simulink model "tut3"  (R2012b)
settings: Solver=ode45  StartTime=0.0  StopTime=8192  RelTol=1e-3
undefined symbols (not defined in the file): gcbh, pfb_coeff_gen_calc, xlBlockLoadCallback
libraries: xbsIndex_r4 x2165, casper_library_misc x93, casper_library_delays x38, xps_library x10, xbsReplacements_r4 x2, casper_library_pfbs x2, simulink x1, casper_library_ffts_twiddle x1, casper_library_reorder x1
(part 17 of 31)

== system tut3/fft_wideband_real/fft_direct/butterfly1_1/twiddle_general_4mult/coeff_gen ==
  rst : Inport
  Counter : xbsIndex_r4/Counter  cnt_type=Free Running  cnt_to=Inf  operation=Up  start_count=0  cnt_by_val=1  arith_type=Unsigned  n_bits=10  bin_pt=0  load_pin=off  rst=on  en=off  explicit_period=on  period=1  dbl_ovrd=off  use_behavioral_HDL=off  implementation=Fabric  block_type=counter
  ROM : xbsIndex_r4/ROM  depth=1024  initVector="[1                                      1                     0.9999847412109375                     0.9999542236328125                     0.9999237060546875                        0.9998779296875                     0.9998321533203125                     0.9997711181640625                       0.99969482421875                     0.9996185302734375                     0.9995269775390625                     0.9994354248046875                       0.99932861328125                       0.99920654296875                       0.99908447265625                     0.9989471435546875                     0.9987945556640625                     0.9986419677734375                       0.99847412109375                     0.9983062744140625                     0.9981231689453125                        0.9979248046875                     0.9977264404296875                     0.9975128173828125                      0.997283935546875                     0.9970550537109375                         0.996826171875                     0.9965667724609375                      0.996307373046875                     0.9960479736328125                     0.9957733154296875                        0.9954833984375                       0.99517822265625                         0.994873046875                       0.99456787109375                     0.9942474365234375                     0.9939117431640625                      0.993560791015625                     0.9932098388671875                     0.9928436279296875                     0.9924774169921875                      0.992095947265625                     0.9917144775390625                     0.9913177490234375                       0.99090576171875                         0.990478515625                       0.99005126953125                        0.9896240234375                     0.9891815185546875                     0.9887237548828125                      0.988250732421875                     0.9877777099609375                           0.9873046875                          0.98681640625                     0.9863128662109375                     0.9857940673828125                     0.9852752685546875                        0.9847412109375                     0.9842071533203125                     0.9836578369140625                     0.9831085205078125                        0.9825439453125                      0.981964111328125                       0.98138427734375                     0.9807891845703125                     0.9801788330078125                     0.9795684814453125                       0.97894287109375                     0.9783172607421875                     0.9776763916015625                     0.9770355224609375                     0.9763641357421875                        0.9757080078125                     0.9750213623046875                      0.974334716796875                     0.9736480712890625                     0.9729461669921875                       0.97222900390625                       0.97149658203125                     0.9707794189453125                       0.97003173828125                     0.9692840576171875                     0.9685211181640625                     0.9677581787109375                       0.96697998046875                        0.9661865234375                       0.96539306640625                     0.9645843505859375                      0.963775634765625                       0.96295166015625                      0.962127685546875                      0.961273193359375                     0.9604339599609375                      0.959564208984375                      0.958709716796875                       0.95782470703125                      0.956939697265625                     0.9560394287109375                       0.95513916015625                        0.9542236328125                       0.95330810546875                     0.9523773193359375                     0.9514312744140625 ...(+35900 chars)]"  distributed_mem=Block RAM  rst=off  init_reg=0  en=off  latency=2  gui_display_data_type=Fixed-point  arith_type="Signed  (2's comp)"  n_bits=18  bin_pt=16  preci_type=Single  exp_width=8  frac_width=24  dbl_ovrd=off  optimize=Area  use_rpm=on  block_type=sprom
  ROM1 : xbsIndex_r4/ROM  depth=1024  initVector="[0                    -0.0030670166015625                     -0.006134033203125                    -0.0092010498046875                      -0.01226806640625                    -0.0153350830078125                     -0.018402099609375                    -0.0214691162109375                       -0.0245361328125                    -0.0276031494140625                     -0.030670166015625                    -0.0337371826171875                      -0.03680419921875                    -0.0398712158203125                     -0.042938232421875                    -0.0460052490234375                        -0.049072265625                    -0.0521392822265625                    -0.0551910400390625                     -0.058258056640625                    -0.0613250732421875                    -0.0643768310546875                      -0.06744384765625                    -0.0705108642578125                    -0.0735626220703125                     -0.076629638671875                     -0.079681396484375                     -0.082733154296875                    -0.0858001708984375                    -0.0888519287109375                    -0.0919036865234375                        -0.094970703125                       -0.0980224609375                         -0.10107421875                       -0.1041259765625                        -0.107177734375                       -0.1102294921875                    -0.1132659912109375                    -0.1163177490234375                    -0.1193695068359375                     -0.122406005859375                     -0.125457763671875                    -0.1284942626953125                    -0.1315460205078125                      -0.13458251953125                    -0.1376190185546875                     -0.140655517578125                    -0.1436920166015625                        -0.146728515625                    -0.1497650146484375                     -0.152801513671875                      -0.15582275390625                    -0.1588592529296875                    -0.1618804931640625                       -0.1649169921875                     -0.167938232421875                      -0.17095947265625                     -0.173980712890625                        -0.177001953125                     -0.180023193359375                      -0.18304443359375                    -0.1860504150390625                    -0.1890716552734375                      -0.19207763671875                    -0.1950836181640625                    -0.1981048583984375                      -0.20111083984375                          -0.2041015625                    -0.2071075439453125                     -0.210113525390625                     -0.213104248046875                    -0.2161102294921875                    -0.2191009521484375                    -0.2220916748046875                    -0.2250823974609375                    -0.2280731201171875                    -0.2310638427734375                     -0.234039306640625                     -0.237030029296875                    -0.2400054931640625                      -0.24298095703125                    -0.2459564208984375                     -0.248931884765625                      -0.25189208984375                    -0.2548675537109375                    -0.2578277587890625                    -0.2607879638671875                    -0.2637481689453125                    -0.2667083740234375                    -0.2696685791015625                    -0.2726287841796875                      -0.27557373046875                    -0.2785186767578125                     -0.281463623046875                    -0.2844085693359375                        -0.287353515625                        -0.290283203125                        -0.293212890625                    -0.2961578369140625                        -0.299072265625                        -0.302001953125                        -0.304931640625                    -0.3078460693359375 ...(+35900 chars)]"  distributed_mem=Block RAM  rst=off  init_reg=0  en=off  latency=2  gui_display_data_type=Fixed-point  arith_type="Signed  (2's comp)"  n_bits=18  bin_pt=16  preci_type=Single  exp_width=8  frac_width=24  dbl_ovrd=off  optimize=Area  use_rpm=on  block_type=sprom
  Slice : xbsIndex_r4/Slice  nbits=10  boolean_output=off  mode=Upper Bit Location + Width  bit1=0  base1=MSB of Input  bit0=0  base0=LSB of Input  dbl_ovrd=off  block_type=slice
  ri_to_c : casper_library_misc/ri_to_c
  w : Outport
  wires:
  ri_to_c/1 -> w/1
  rst/1 -> Counter/1
  Counter/1 -> Slice/1
  Slice/1 -> ROM/1, ROM1/1
  ROM/1 -> ri_to_c/1
  ROM1/1 -> ri_to_c/2
